simulink model "linear_controller"  (R2024b)
settings: Solver=VariableStepAuto  StartTime=0.0  StopTime=25  RelTol=1e-3
libraries: roblocks x1

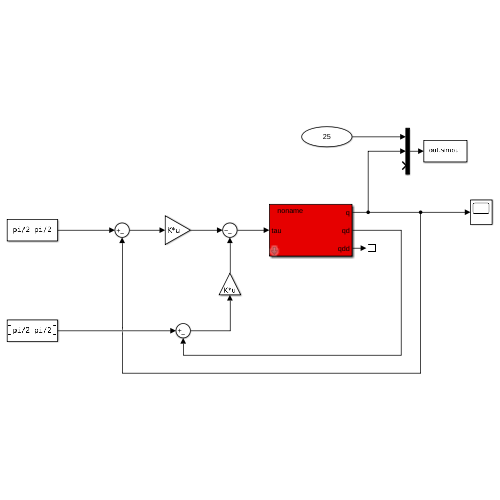
[thumbnail: Simulink's stored preview of the top-level diagram]
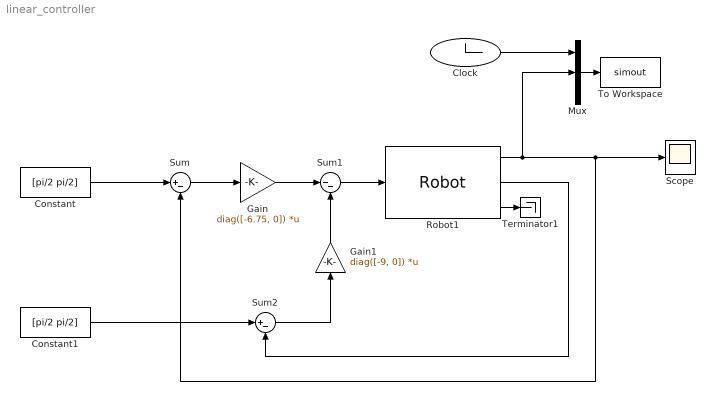
== system linear_controller ==
  Clock : Clock
  Constant : Constant  Value=[pi/2 pi/2]
  Constant1 : Constant  Value=[pi/2 pi/2]
  Gain : Gain  Gain=diag([-6.75, 0])  Multiplication=Matrix(K*u)
  Gain1 : Gain  Gain=diag([-9, 0])  Multiplication=Matrix(K*u)
  Mux : Mux  Inputs=3
  Robot1 : roblocks/Robot  robot=robot  q0=[0 0 0 0 0 0]
  Scope : Scope
  Sum : Sum  Inputs=|+-
  Sum1 : Sum  Inputs=|--
  Sum2 : Sum  Inputs=|+-
  Terminator1 : Terminator
  To Workspace : ToWorkspace  VariableName=simout  SampleTime=-1
  wires:
  Sum/1 -> Gain/1
  Gain1/1 -> Sum1/2
  Sum2/1 -> Gain1/1
  Clock/1 -> Mux/1
  Mux/1 -> To Workspace/1
  Gain/1 -> Sum1/1
  Constant/1 -> Sum/1
  Constant1/1 -> Sum2/1
  Robot1/2 -> Sum2/2
  Robot1/1 -> Mux/2, Scope/1, Sum/2
  Robot1/3 -> Terminator1/1
  Sum1/1 -> Robot1/1
